simulink model "stateFeedbackRobustControllerModel"  (R2021a)
settings: Solver=VariableStepAuto  StartTime=0.0  StopTime=10.0  RelTol=1e-3
settings Model: Creator=krzys  LastModifiedBy=krzys

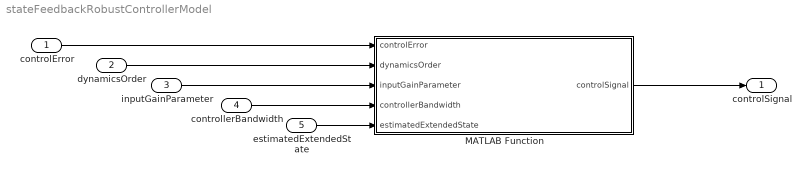
== system stateFeedbackRobustControllerModel ==
  controlError : Inport
  dynamicsOrder : Inport  Port=2
  inputGainParameter : Inport  Port=3
  controllerBandwidth : Inport  Port=4
  estimatedExtendedState : Inport  Port=5
  MATLAB Function : MATLAB Function  TreatAsAtomicUnit=on
  controlSignal : Outport
  wires:
  dynamicsOrder/1 -> MATLAB Function/2(dynamicsOrder)
  inputGainParameter/1 -> MATLAB Function/3(inputGainParameter)
  controllerBandwidth/1 -> MATLAB Function/4(controllerBandwidth)
  estimatedExtendedState/1 -> MATLAB Function/5(estimatedExtendedState)
  MATLAB Function/1(controlSignal) -> controlSignal/1
  controlError/1 -> MATLAB Function/1(controlError)

== matlab function stateFeedbackRobustControllerModel/MATLAB Function ==
  data: controlError input; dynamicsOrder input; controlSignal output; inputGainParameter input; controllerBandwidth input; estimatedExtendedState input
function controlSignal = fcn(controlError,...
        dynamicsOrder,...
        inputGainParameter,...
        controllerBandwidth,...
        estimatedExtendedState)
   
    K = calculateControllerGain(controllerBandwidth, dynamicsOrder);
    
    controlSignal = 1/inputGainParameter * (estimatedExtendedState(end) + ...
            K * [controlError; estimatedExtendedState(2:end-1)]);
end

function controllerGain = calculateControllerGain(controllerBandwidth, dynamicsOrder)
    extendedControllerGain = poly(-controllerBandwidth * ones(1, dynamicsOrder));
    controllerGain = extendedControllerGain(2:end);
end
